simulink model "msd"  (R2025b)
settings: Solver=VariableStepAuto  StartTime=0.0  StopTime=50  RelTol=1e-6
settings Model: Creator=Rocksmithed  LastModifiedBy=garellan
settings SolverCC: AlgebraicLoopSolver=TrustRegion
settings DebuggingCC: UnconnectedInputMsg=warning  UnconnectedOutputMsg=warning  UnconnectedLineMsg=warning
settings ModelReferenceCC: EnableRefExpFcnMdlSchedulingChecks=on
settings RTWCC: GPUComputeCapability=3.5  DLArmComputeVersion=19.05

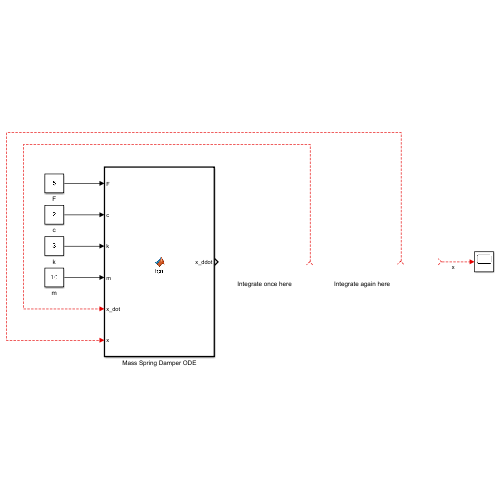
[thumbnail: Simulink's stored preview of the top-level diagram]
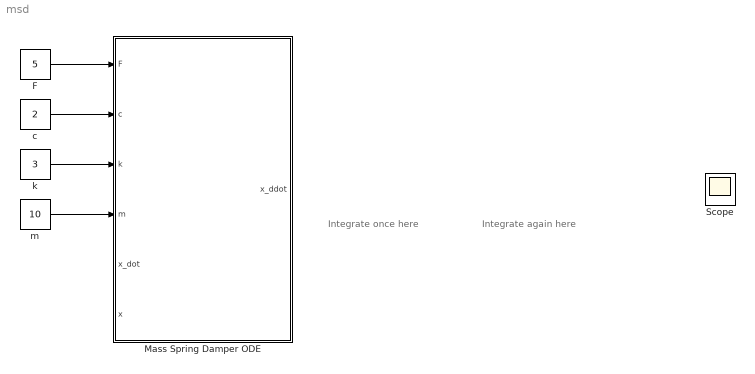
== system msd ==
  note: Integrate once here
  note: Integrate again here
  F : Constant  Value=5
  Mass Spring Damper ODE : MATLAB Function  TreatAsAtomicUnit=on
  Scope : Scope
      settings: ActiveDisplayYMinimum=-0.32393770210017747  ActiveDisplayYMaximum=2.9154393189015977
  c : Constant  Value=2
  k : Constant  Value=3
  m : Constant  Value=10
  wires:
  F/1 -> Mass Spring Damper ODE/1(F)
  c/1 -> Mass Spring Damper ODE/2(c)
  k/1 -> Mass Spring Damper ODE/3(k)
  m/1 -> Mass Spring Damper ODE/4(m)
  ? -> Mass Spring Damper ODE/5(x_dot)
  ? -> Scope/1  "x"
  ? -> Mass Spring Damper ODE/6(x)

== matlab function msd/Mass Spring Damper ODE ==
  data: F input; x_ddot output; c input; k input; m input; x_dot input; x input
function x_ddot = fcn(F,c,k,m,x_dot,x)

   % Write your expression for x_ddot here in terms of the inputs
   x_ddot = -(-F+c.*x_dot+k.*x)./m;
end
